simulink model "Local_Oscillator"  (R2017a)
settings: Solver=VariableStepAuto  StartTime=0.0  StopTime=0.001  RelTol=1e-3
settings Model: Creator=Alam  LastModifiedBy=Alam

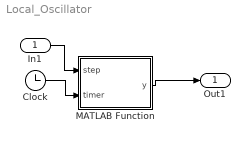
== system Local_Oscillator ==
  In1 : Inport
  Clock : Clock
  MATLAB Function : MATLAB Function  TreatAsAtomicUnit=on  SystemSampleTime=2.61834939e-8
  Out1 : Outport
  wires:
  MATLAB Function/1(y) -> Out1/1
  In1/1 -> MATLAB Function/1(step)
  Clock/1 -> MATLAB Function/2(timer)

== matlab function Local_Oscillator/MATLAB Function ==
  data: y output; step input; timer input
function y = Local_Oscillator(step, timer)
f = step*500+9548000;
y = exp(1i*(2*pi*f*timer));
